simulink model "Control_Bilateral"  (R2015b)
settings: Solver=VariableStepAuto  StartTime=0.0  StopTime=50  RelTol=1e-3
values from neighbouring files (symbols this model uses):
  b = 0.20    (= 0.2)    [Bilateral.m]
  Be = 0.25    [Bilateral.m]
  Bm = 20    [Bilateral.m]    (also in matlab-DESKTOP-P6EB44P.mat; matlab.mat)
  Bs = 20    [Bilateral.m]    (also in matlab-DESKTOP-P6EB44P.mat; matlab.mat)
  Ke = 0.25    [Bilateral.m]    (also in matlab-DESKTOP-P6EB44P.mat = 30)
  Kf = 100    [Bilateral.m]    (also in matlab-DESKTOP-P6EB44P.mat; matlab.mat)
  Kh = 0.25 * i    [Bilateral.m]    (also in matlab-DESKTOP-P6EB44P.mat = 0; matlab.mat = 100)
  Kpm = 0.1    [Bilateral.m]    (also in matlab-DESKTOP-P6EB44P.mat = 0.25)
  Kps = 100    [Bilateral.m]    (also in matlab-DESKTOP-P6EB44P.mat)
  Mm = 1    [Bilateral.m]    (also in matlab-DESKTOP-P6EB44P.mat; matlab.mat)
  Ms = 1    [Bilateral.m]    (also in matlab-DESKTOP-P6EB44P.mat; matlab.mat)
  S = 1    [Bilateral.m]
  Td = 2.0    (= 2)    [Bilateral.m]    (also in matlab-DESKTOP-P6EB44P.mat = 0.001)
settings Model: Creator=Jcama  LastModifiedBy=Jcama

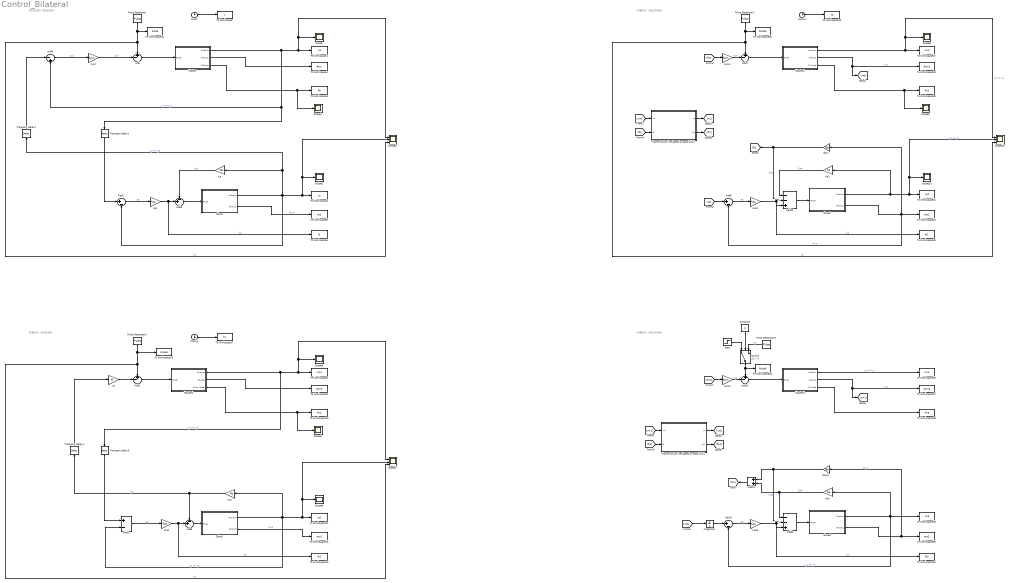
== system Control_Bilateral ==
  note: POSICIÓN - POSICIÓN
  note: FUERZA - POSICIÓN
  note: FUERZA - VELOCIDAD
  note: FUERZA - VELOCIDAD
  Add{,1,7,11} (4 alike) : Sum  Inputs=+-|
  Add10 : Sum  Inputs=--+|
  Add12 : Sum  Inputs=|+-
  Add13 : Sum
  Add2 : Sum  Inputs=|+-
  Add3 : Sum  Inputs=+-
  Add4 : Sum  Inputs=|-+
  Add5 : Sum  Inputs=-+|
  Add6 : Sum  Inputs=-+|
  Add8 : Sum  Inputs=|+-
  Add9 : Sum  Inputs=--+|
  Clock : Clock
  Clock1 : Clock
  Clock2 : Clock
  Constant : Constant  Value=S
  Gain : Gain  Gain=Be
  Gain1 : Gain  Gain=Be
  Integrator : Integrator
  Ke{,1..3} (4 alike) : Gain  Gain=Ke
  Kf : Gain  Gain=Kf
  Kpm : Gain  Gain=Kpm
  Kpm1 : Gain  Gain=Kpm
  Kpm2 : Gain  Gain=Kpm
  Kps{,1..3} (4 alike) : Gain  Gain=Kps
  Master : Subsystem
  Master1 : Subsystem
  Master2 : Subsystem
  Master3 : Subsystem
  Pulse Generator{,1..3} (4 alike) : DiscretePulseGenerator  PulseType=Time based  Period=10  PulseWidth=10
  Scope{,1..2,4..6,8..10} (9 alike) : Scope
  Scope11 : Scope  NumInputPorts=3
  Scope3 : Scope  NumInputPorts=3
  Scope7 : Scope  NumInputPorts=3
  Slave : Subsystem
  Slave1 : Subsystem
  Slave2 : Subsystem
  Slave3 : Subsystem
  Step : Step  Time=2  Before=1  After=0  SampleTime=0
  Switch : Switch  Criteria=u2 > Threshold
  To Workspace : ToWorkspace  VariableName=t  SaveFormat=Timeseries  SampleTime=-1
  To Workspace1 : ToWorkspace  VariableName=xm  SaveFormat=Timeseries  SampleTime=-1
  To Workspace10 : ToWorkspace  VariableName=fm1  SaveFormat=Timeseries  SampleTime=-1
  To Workspace11 : ToWorkspace  VariableName=xs1  SaveFormat=Timeseries  SampleTime=-1
  To Workspace12 : ToWorkspace  VariableName=dxs1  SaveFormat=Timeseries  SampleTime=-1
  To Workspace13 : ToWorkspace  VariableName=fs1  SaveFormat=Timeseries  SampleTime=-1
  To Workspace14 : ToWorkspace  VariableName=Pulse  SaveFormat=Timeseries  SampleTime=-1
  To Workspace15 : ToWorkspace  VariableName=Pulse1  SaveFormat=Timeseries  SampleTime=-1
  To Workspace16 : ToWorkspace  VariableName=t2  SaveFormat=Timeseries  SampleTime=-1
  To Workspace17 : ToWorkspace  VariableName=xm2  SaveFormat=Timeseries  SampleTime=-1
  To Workspace18 : ToWorkspace  VariableName=Pulse2  SaveFormat=Timeseries  SampleTime=-1
  To Workspace19 : ToWorkspace  VariableName=dxm2  SaveFormat=Timeseries  SampleTime=-1
  To Workspace2 : ToWorkspace  VariableName=dxm  SaveFormat=Timeseries  SampleTime=-1
  To Workspace20 : ToWorkspace  VariableName=fm2  SaveFormat=Timeseries  SampleTime=-1
  To Workspace21 : ToWorkspace  VariableName=xs2  SaveFormat=Timeseries  SampleTime=-1
  To Workspace22 : ToWorkspace  VariableName=dxs2  SaveFormat=Timeseries  SampleTime=-1
  To Workspace23 : ToWorkspace  VariableName=fs2  SaveFormat=Timeseries  SampleTime=-1
  To Workspace25 : ToWorkspace  VariableName=xm3  SaveFormat=Timeseries  SampleTime=-1
  To Workspace26 : ToWorkspace  VariableName=Pulse3  SaveFormat=Timeseries  SampleTime=-1
  To Workspace27 : ToWorkspace  VariableName=dxm3  SaveFormat=Timeseries  SampleTime=-1
  To Workspace28 : ToWorkspace  VariableName=fm3  SaveFormat=Timeseries  SampleTime=-1
  To Workspace29 : ToWorkspace  VariableName=xs3  SaveFormat=Timeseries  SampleTime=-1
  To Workspace3 : ToWorkspace  VariableName=fm  SaveFormat=Timeseries  SampleTime=-1
  To Workspace30 : ToWorkspace  VariableName=dxs3  SaveFormat=Timeseries  SampleTime=-1
  To Workspace31 : ToWorkspace  VariableName=fs3  SaveFormat=Timeseries  SampleTime=-1
  To Workspace4 : ToWorkspace  VariableName=xs  SaveFormat=Timeseries  SampleTime=-1
  To Workspace5 : ToWorkspace  VariableName=dxs  SaveFormat=Timeseries  SampleTime=-1
  To Workspace6 : ToWorkspace  VariableName=fs  SaveFormat=Timeseries  SampleTime=-1
  To Workspace7 : ToWorkspace  VariableName=t1  SaveFormat=Timeseries  SampleTime=-1
  To Workspace8 : ToWorkspace  VariableName=xm1  SaveFormat=Timeseries  SampleTime=-1
  To Workspace9 : ToWorkspace  VariableName=dxm1  SaveFormat=Timeseries  SampleTime=-1
  Transmission line based on passivity1 : Subsystem
  Transmission line based on passivity2 : Subsystem
  Transport Delay{1..4} (4 alike) : TransportDelay  DelayTime=Td
  wires:
  Clock/1 -> To Workspace/1
  Pulse Generator/1 -> To Workspace14/1, Scope3/3, Add/1  "f_h"
  Master/1(Position) -> Add4/2, Transport Delay1/1, Scope/1, Scope3/1, To Workspace1/1  "x_m = x_h"
  Slave/1(Position) -> Add2/2, Transport Delay2/1, Ke/1, Scope3/2, Scope2/1, To Workspace4/1  "x_s  = x_e"
  Add4/1 -> Kpm/1  "e_p"
  Kpm/1 -> Add/2  "f_m"
  Add/1 -> Master/1(Force)
  Master/2(Velocity) -> To Workspace2/1
  Master/3(Kf Force) -> Scope1/1, To Workspace3/1
  Slave/2(Velocity) -> To Workspace5/1  "dx_s"
  Add2/1 -> Kps/1  "ep"
  Kps/1 -> Add5/2, To Workspace6/1  "f_s"
  Add5/1 -> Slave/1(Force)
  Ke/1 -> Add5/1  "f_e"
  Clock1/1 -> To Workspace7/1
  Pulse Generator1/1 -> To Workspace15/1, Scope7/3, Add1/1  "f_h"
  Master1/1(Position) -> Scope4/1, Scope7/1, To Workspace8/1, Transport Delay3/1  "x_m = x_h"
  Slave1/1(Position) -> Ke1/1, Scope7/2, Scope6/1, To Workspace11/1, Add3/2  "x_s  = x_e"
  Add1/1 -> Master1/1(Force)
  Master1/2(Velocity) -> To Workspace9/1
  Master1/3("  Entry Force") -> Scope5/1, To Workspace10/1
  Slave1/2(Velocity) -> To Workspace12/1  "dx_s"
  Add3/1 -> Kps1/1  "ep"
  Kps1/1 -> Add6/2, To Workspace13/1  "f_s"
  Transport Delay1/1 -> Add2/1
  Transport Delay3/1 -> Add3/1
  Transport Delay4/1 -> Kf/1
  Add6/1 -> Slave1/1(Force)
  Ke1/1 -> Transport Delay4/1, Add6/1  "f_e"
  Transport Delay2/1 -> Add4/1
  Kf/1 -> Add1/2
  Clock2/1 -> To Workspace16/1
  Pulse Generator2/1 -> To Workspace18/1, Scope11/3, Add7/1  "f_h"
  Master2/1(Position) -> Scope8/1, Scope11/1, To Workspace17/1  "x_m = x_h"
  Slave2/1(Position) -> Ke2/1, To Workspace21/1, Scope11/2, Scope10/1  "x_s  = x_e"
  Kpm1/1 -> Add7/2  "f_m"
  Add7/1 -> Master2/1(Force)
  Master2/2(Velocity) -> [vm], To Workspace19/1  "v_m"
  Master2/3(Kf Force) -> Scope9/1, To Workspace20/1
  Slave2/2(Velocity) -> Add8/2, Gain/1, To Workspace22/1  "dx_s"
  Add8/1 -> Kps2/1  "ep"
  Kps2/1 -> Add10/3, To Workspace23/1  "f_s"
  Add10/1 -> Slave2/1(Force)
  Ke2/1 -> Add10/1  "f_ke"
  [vs] -> Add8/1
  [fm] -> Kpm1/1
  Gain/1 -> [fs], Add10/2  "f_be"
  Master3/1(Position) -> To Workspace25/1  "x_m = x_h"
  Slave3/1(Position) -> Add12/2, Ke3/1, To Workspace29/1  "x_s  = x_e"
  Kpm2/1 -> Add11/2  "f_m"
  Add11/1 -> Master3/1(Force)
  Master3/2(Velocity) -> [vm1], To Workspace27/1  "v_m"
  Master3/3(Kf Force) -> To Workspace28/1
  Slave3/2(Velocity) -> Gain1/1, To Workspace30/1  "dx_s"
  Add12/1 -> Kps3/1  "ep"
  Kps3/1 -> Add9/3, To Workspace31/1  "f_s"
  Add9/1 -> Slave3/1(Force)
  Ke3/1 -> Add9/1, Add13/2  "f_ke"
  [vm1] -> Transmission line based on passivity1/1(vm)
  [fs1] -> Transmission line based on passivity1/2(fs)
  Transmission line based on passivity1/1(vs) -> [vs1]
  Transmission line based on passivity1/2(fm) -> [fm1]
  [vs1] -> Integrator/1
  [fm1] -> Kpm2/1
  Gain1/1 -> Add9/2, Add13/1  "f_be"
  Integrator/1 -> Add12/1
  Add13/1 -> [fs1]
  Pulse Generator3/1 -> Switch/3  "f_h"
  Switch/1 -> Add11/1, To Workspace26/1
  Step/1 -> Switch/1
  Constant/1 -> Switch/2
  [vm] -> Transmission line based on passivity2/1(vm)
  [fs] -> Transmission line based on passivity2/2(fs)
  Transmission line based on passivity2/1(vs) -> [vs]
  Transmission line based on passivity2/2(fm) -> [fm]

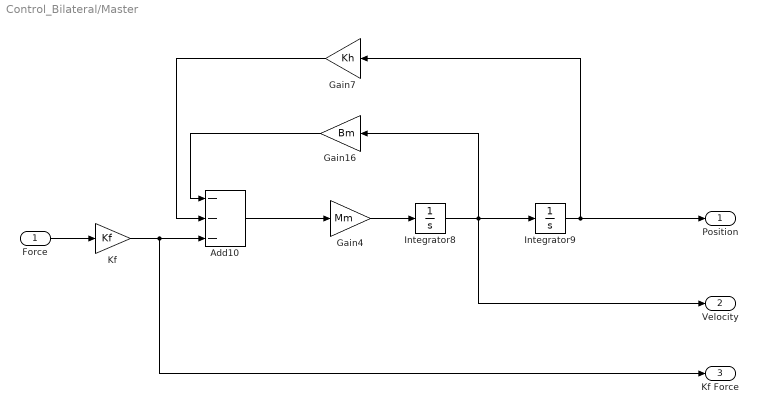
== system Control_Bilateral/Master ==
  Force : Inport
  Add10 : Sum  Inputs=---
  Gain16 : Gain  Gain=Bm
  Gain4 : Gain  Gain=Mm
  Gain7 : Gain  Gain=Kh
  Integrator8 : Integrator
  Integrator9 : Integrator
  Kf : Gain  Gain=Kf
  Position : Outport
  Velocity : Outport  Port=2
  Kf Force : Outport  Port=3
  wires:
  Add10/1 -> Gain4/1
  Gain16/1 -> Add10/1
  Gain7/1 -> Add10/2
  Gain4/1 -> Integrator8/1
  Kf/1 -> Kf Force/1, Add10/3
  Integrator8/1 -> Velocity/1, Gain16/1, Integrator9/1
  Integrator9/1 -> Position/1, Gain7/1
  Force/1 -> Kf/1

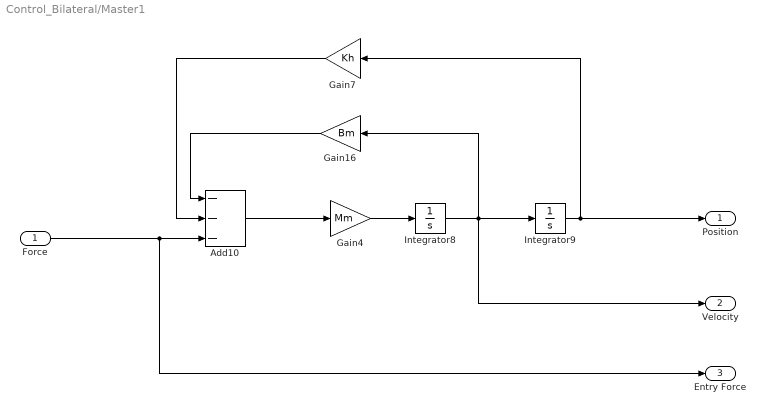
== system Control_Bilateral/Master1 ==
  Force : Inport
  Add10 : Sum  Inputs=---
  Gain16 : Gain  Gain=Bm
  Gain4 : Gain  Gain=Mm
  Gain7 : Gain  Gain=Kh
  Integrator8 : Integrator
  Integrator9 : Integrator
  Position : Outport
  Velocity : Outport  Port=2
  "  Entry Force" : Outport  Port=3
  wires:
  Add10/1 -> Gain4/1
  Gain16/1 -> Add10/1
  Gain7/1 -> Add10/2
  Gain4/1 -> Integrator8/1
  Force/1 -> "  Entry Force"/1, Add10/3
  Integrator8/1 -> Velocity/1, Gain16/1, Integrator9/1
  Integrator9/1 -> Position/1, Gain7/1

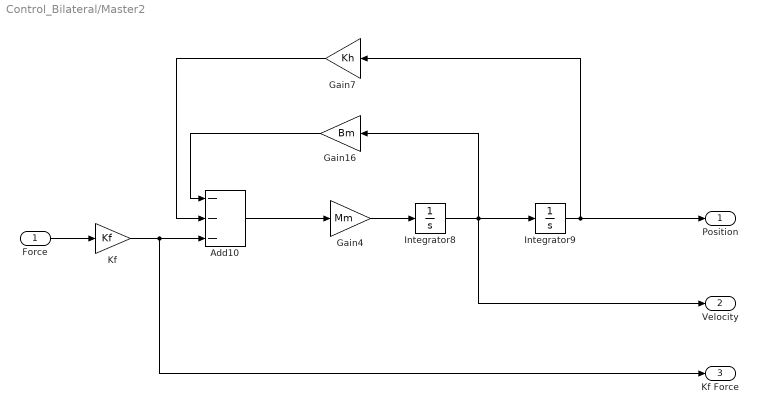
== system Control_Bilateral/Master2 ==
  Force : Inport
  Add10 : Sum  Inputs=---
  Gain16 : Gain  Gain=Bm
  Gain4 : Gain  Gain=Mm
  Gain7 : Gain  Gain=Kh
  Integrator8 : Integrator
  Integrator9 : Integrator
  Kf : Gain  Gain=Kf
  Position : Outport
  Velocity : Outport  Port=2
  Kf Force : Outport  Port=3
  wires:
  Add10/1 -> Gain4/1
  Gain16/1 -> Add10/1
  Gain7/1 -> Add10/2
  Gain4/1 -> Integrator8/1
  Kf/1 -> Kf Force/1, Add10/3
  Integrator8/1 -> Velocity/1, Gain16/1, Integrator9/1
  Integrator9/1 -> Position/1, Gain7/1
  Force/1 -> Kf/1

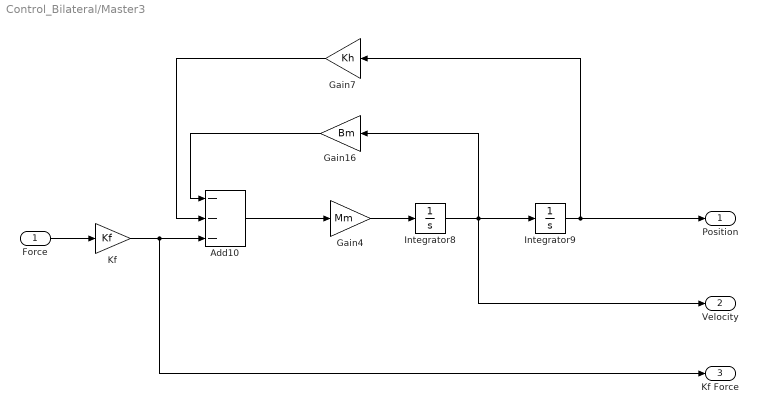
== system Control_Bilateral/Master3 ==
  Force : Inport
  Add10 : Sum  Inputs=---
  Gain16 : Gain  Gain=Bm
  Gain4 : Gain  Gain=Mm
  Gain7 : Gain  Gain=Kh
  Integrator8 : Integrator
  Integrator9 : Integrator
  Kf : Gain  Gain=Kf
  Position : Outport
  Velocity : Outport  Port=2
  Kf Force : Outport  Port=3
  wires:
  Add10/1 -> Gain4/1
  Gain16/1 -> Add10/1
  Gain7/1 -> Add10/2
  Gain4/1 -> Integrator8/1
  Kf/1 -> Kf Force/1, Add10/3
  Integrator8/1 -> Velocity/1, Gain16/1, Integrator9/1
  Integrator9/1 -> Position/1, Gain7/1
  Force/1 -> Kf/1

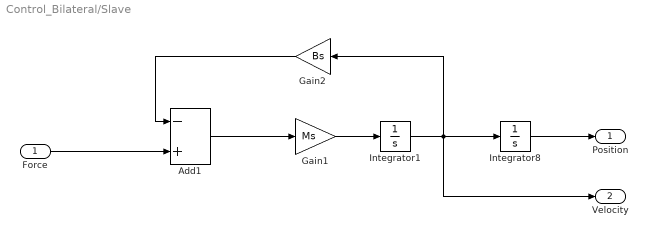
== system Control_Bilateral/Slave ==
  Force : Inport
  Add1 : Sum  Inputs=-+
  Gain1 : Gain  Gain=Ms
  Gain2 : Gain  Gain=Bs
  Integrator1 : Integrator
  Integrator8 : Integrator
  Position : Outport
  Velocity : Outport  Port=2
  wires:
  Integrator8/1 -> Position/1
  Gain2/1 -> Add1/1
  Integrator1/1 -> Velocity/1, Gain2/1, Integrator8/1
  Gain1/1 -> Integrator1/1
  Add1/1 -> Gain1/1
  Force/1 -> Add1/2

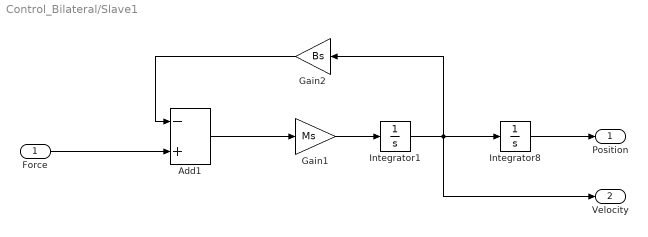
== system Control_Bilateral/Slave1 ==
  Force : Inport
  Add1 : Sum  Inputs=-+
  Gain1 : Gain  Gain=Ms
  Gain2 : Gain  Gain=Bs
  Integrator1 : Integrator
  Integrator8 : Integrator
  Position : Outport
  Velocity : Outport  Port=2
  wires:
  Integrator8/1 -> Position/1
  Gain2/1 -> Add1/1
  Integrator1/1 -> Velocity/1, Gain2/1, Integrator8/1
  Gain1/1 -> Integrator1/1
  Add1/1 -> Gain1/1
  Force/1 -> Add1/2

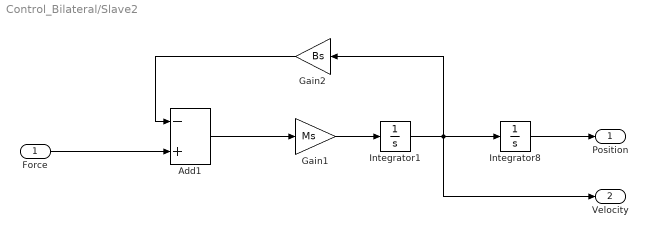
== system Control_Bilateral/Slave2 ==
  Force : Inport
  Add1 : Sum  Inputs=-+
  Gain1 : Gain  Gain=Ms
  Gain2 : Gain  Gain=Bs
  Integrator1 : Integrator
  Integrator8 : Integrator
  Position : Outport
  Velocity : Outport  Port=2
  wires:
  Integrator8/1 -> Position/1
  Gain2/1 -> Add1/1
  Integrator1/1 -> Velocity/1, Gain2/1, Integrator8/1
  Gain1/1 -> Integrator1/1
  Add1/1 -> Gain1/1
  Force/1 -> Add1/2

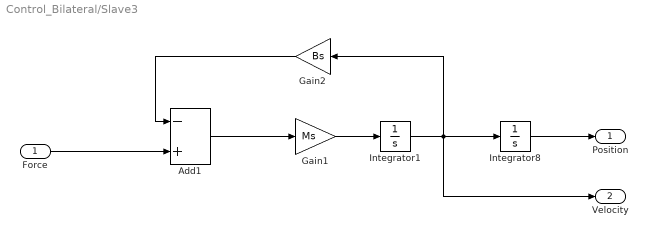
== system Control_Bilateral/Slave3 ==
  Force : Inport
  Add1 : Sum  Inputs=-+
  Gain1 : Gain  Gain=Ms
  Gain2 : Gain  Gain=Bs
  Integrator1 : Integrator
  Integrator8 : Integrator
  Position : Outport
  Velocity : Outport  Port=2
  wires:
  Integrator8/1 -> Position/1
  Gain2/1 -> Add1/1
  Integrator1/1 -> Velocity/1, Gain2/1, Integrator8/1
  Gain1/1 -> Integrator1/1
  Add1/1 -> Gain1/1
  Force/1 -> Add1/2

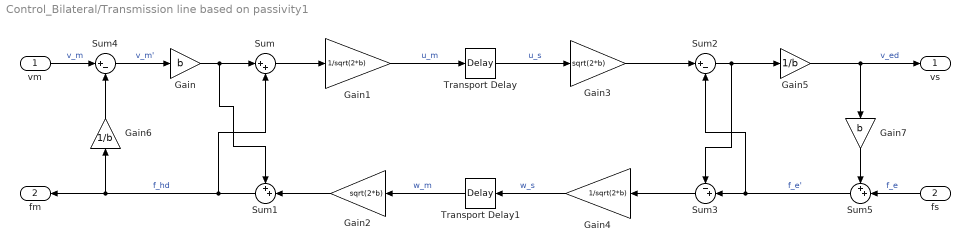
== system Control_Bilateral/Transmission line based on passivity1 ==
  vm : Inport
  fs : Inport  Port=2
  Gain : Gain  Gain=b
  Gain1 : Gain  Gain=1/sqrt(2*b)
  Gain2 : Gain  Gain=sqrt(2*b)
  Gain3 : Gain  Gain=sqrt(2*b)
  Gain4 : Gain  Gain=1/sqrt(2*b)
  Gain5 : Gain  Gain=1/b
  Gain6 : Gain  Gain=1/b
  Gain7 : Gain  Gain=b
  Sum : Sum  Inputs=|++
  Sum1 : Sum  Inputs=++|
  Sum2 : Sum  Inputs=|+-
  Sum3 : Sum  Inputs=-+|
  Sum4 : Sum  Inputs=|+-
  Sum5 : Sum  Inputs=++|
  Transport Delay : TransportDelay  DelayTime=Td
  Transport Delay1 : TransportDelay  DelayTime=Td
  vs : Outport
  fm : Outport  Port=2
  wires:
  Gain/1 -> Sum/1, Sum1/1
  Sum/1 -> Gain1/1
  Gain2/1 -> Sum1/2
  Transport Delay1/1 -> Gain2/1  "w_m"
  Gain1/1 -> Transport Delay/1  "u_m"
  Transport Delay/1 -> Gain3/1  "u_s"
  Gain4/1 -> Transport Delay1/1  "w_s"
  Gain3/1 -> Sum2/1
  Sum3/1 -> Gain4/1
  Sum2/1 -> Gain5/1, Sum3/1
  Gain5/1 -> Gain7/1, vs/1  "v_ed"
  vm/1 -> Sum4/1  "v_m"
  Sum4/1 -> Gain/1  "v_m'"
  Gain6/1 -> Sum4/2
  Sum1/1 -> Gain6/1, fm/1, Sum/2  "f_hd"
  fs/1 -> Sum5/2  "f_e"
  Sum5/1 -> Sum2/2, Sum3/2  "f_e'"
  Gain7/1 -> Sum5/1

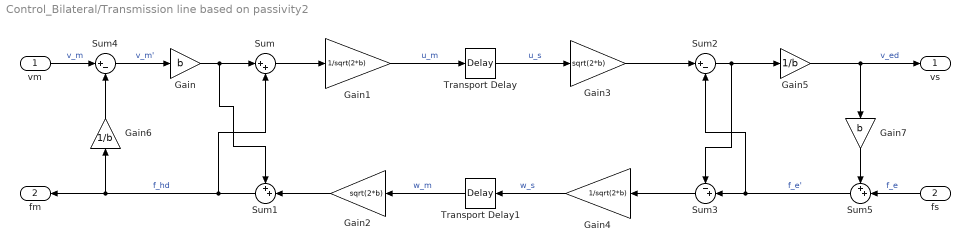
== system Control_Bilateral/Transmission line based on passivity2 ==
  vm : Inport
  fs : Inport  Port=2
  Gain : Gain  Gain=b
  Gain1 : Gain  Gain=1/sqrt(2*b)
  Gain2 : Gain  Gain=sqrt(2*b)
  Gain3 : Gain  Gain=sqrt(2*b)
  Gain4 : Gain  Gain=1/sqrt(2*b)
  Gain5 : Gain  Gain=1/b
  Gain6 : Gain  Gain=1/b
  Gain7 : Gain  Gain=b
  Sum : Sum  Inputs=|++
  Sum1 : Sum  Inputs=++|
  Sum2 : Sum  Inputs=|+-
  Sum3 : Sum  Inputs=-+|
  Sum4 : Sum  Inputs=|+-
  Sum5 : Sum  Inputs=++|
  Transport Delay : TransportDelay  DelayTime=Td
  Transport Delay1 : TransportDelay  DelayTime=Td
  vs : Outport
  fm : Outport  Port=2
  wires:
  Gain/1 -> Sum/1, Sum1/1
  Sum/1 -> Gain1/1
  Gain2/1 -> Sum1/2
  Transport Delay1/1 -> Gain2/1  "w_m"
  Gain1/1 -> Transport Delay/1  "u_m"
  Transport Delay/1 -> Gain3/1  "u_s"
  Gain4/1 -> Transport Delay1/1  "w_s"
  Gain3/1 -> Sum2/1
  Sum3/1 -> Gain4/1
  Sum2/1 -> Gain5/1, Sum3/1
  Gain5/1 -> Gain7/1, vs/1  "v_ed"
  vm/1 -> Sum4/1  "v_m"
  Sum4/1 -> Gain/1  "v_m'"
  Gain6/1 -> Sum4/2
  Sum1/1 -> Gain6/1, fm/1, Sum/2  "f_hd"
  fs/1 -> Sum5/2  "f_e"
  Sum5/1 -> Sum2/2, Sum3/2  "f_e'"
  Gain7/1 -> Sum5/1
